simulink model "model_sysid_admittance"  (R2016b)
settings: Solver=FixedStepDiscrete  StartTime=0.0  StopTime=inf  FixedStep=sampleTime  RelTol=1e-3
PostLoadFcn:
  | % load model parameters
  | % pname = fileparts(get_param('model_base_bros','filename'));
  | % run([pname  '\parameters_base_model_bros.m']);
  | parameters_sysid_admittance;
  | 
  | % set requested state
  | set_param('model_sysid_admittance/Requested state','Value',num2str(0));
InitFcn:
  | % load model parameters
  | % pname = fileparts(get_param('model_base_bros','filename'));
  | % run([pname  '\parameters_base_model_bros.m']);
  | parameters_sysid_admittance;
  | 
  | % set requested state
  | set_param('model_sysid_admittance/Requested state','Value',num2str(0));
StartFcn:
  | parameters_sysid_admittance;
  | 
  | % set requested state
  | set_param('model_sysid_admittance/Requested state','Value',num2str(0));
values from neighbouring files (symbols this model uses):
  Ax = [0.00153392997769 0.00153392997769 0.00153392997769 0.00153392997769 0.00153392997769 0.00153392997769 0.00153392997769 0.00153392997769 0.00153392997769 0.00153392997769 0.00153392997769 0.00153392997769 ... (25 elements, 25x1)]    [data_inputsignal_admittance_100Hz.mat]
  Ay = [0.00153392997769 0.00153392997769 0.00153392997769 0.00153392997769 0.00153392997769 0.00153392997769 0.00153392997769 0.00153392997769 0.00153392997769 0.00153392997769 0.00153392997769 0.00153392997769 ... (25 elements, 25x1)]    [data_inputsignal_admittance_100Hz.mat]
  Lb = 0.07    [model_affc_parameters.m]    (also in parameters_sysid.m; parameters_sysid_admittance.m)
  Lf = 0.238    [model_affc_parameters.m]    (also in parameters_sysid.m; parameters_sysid_admittance.m)
  Lu = 0.153    [model_affc_parameters.m]    (also in parameters_sysid.m; parameters_sysid_admittance.m)
  nx = [5 7 11 13 17 23 29 37 47 61 79 103 ... (25 elements, 25x1)]    [data_inputsignal_admittance_100Hz.mat]
  ny = [3 8 10 14 19 24 31 41 53 67 83 107 ... (25 elements, 25x1)]    [data_inputsignal_admittance_100Hz.mat]
  phx = [1.20009664335 1.06282811403 1.3892882876 -0.190948998613 4.36135308948 3.55125265665 -1.29943418487 -0.0100316069113 1.01892216761 0.472716168264 1.16765179672 3.48382334533 ... (25 elements, 25x1)]    [data_inputsignal_admittance_100Hz.mat]
  phy = [4.61290873425 3.09865303555 -1.33576318949 -0.454866147562 0.315570179572 -1.54269258334 1.9231806523 3.28701306913 -0.551495079422 2.37779557242 1.0737629469 -1.42157877686 ... (25 elements, 25x1)]    [data_inputsignal_admittance_100Hz.mat]
  sampleTime = 0.001    [model_affc_parameters.m]    (also in parameters_sysid.m; parameters_sysid_admittance.m)
  Tm = 12    [data_inputsignal.mat]    (also in data_inputsignal_100Hz.mat; data_inputsignal_100Hz_n40.mat; data_inputsignal_150Hz_n50.mat; data_inputsignal_50Hz.mat)
undefined symbols (not defined in the file or in its folder): BROS3
libraries: simulink x14, LibraryFM x7, VariousBlocksLibrary x6, simulink_extras x1
(part 2 of 2)

== system model_sysid_admittance/Robot1/DataFromEtherCAT/Calculate Arrange Joint and Op Space/forward kinematics1 ==
  JointPosition_rad : Inport  PortDimensions=[2 1]
  JointVelocity_rads : Inport  Port=2  PortDimensions=[2 1]
  JointAcceleration_rads2 : Inport  Port=3  PortDimensions=[2 1]
  Je : MATLAB Function  TreatAsAtomicUnit=on
  Jedot : MATLAB Function  TreatAsAtomicUnit=on
  Product : Product  Multiplication=Matrix(*)
  calculate xddot : MATLAB Function  TreatAsAtomicUnit=on
  forward kinematics : MATLAB Function  TreatAsAtomicUnit=on
  x : Outport
  xdot : Outport  Port=2
  xddot : Outport  Port=3
  J : Outport  Port=4
  Jdot : Outport  Port=5
  wires:
  JointPosition_rad/1 -> forward kinematics/1(q), Jedot/1(q), Je/1(q)
  Je/1(Je) -> calculate xddot/3(J), Product/1, J/1
  JointVelocity_rads/1 -> calculate xddot/2(qdot), Product/2, Jedot/2(qdot)
  Jedot/1(Jedot) -> calculate xddot/4(Jdot), Jdot/1
  Product/1 -> xdot/1
  forward kinematics/1(x) -> x/1
  calculate xddot/1(xddot) -> xddot/1
  JointAcceleration_rads2/1 -> calculate xddot/1(qddot)

== matlab function model_sysid_admittance/Experiment & Haptics1/Admittance3/MATLAB Function ==
  data: t input; p output; nx parameter; Ax parameter; phx parameter; v output; a output; Tm parameter; ny parameter; Ay parameter; phy parameter
function [p,v,a] = fcn(t, nx, Ax, phx, Tm, ny, Ay, phy)
%#codegen

dw = 2*pi/Tm;
wx = nx*dw;
wy = ny*dw;

x = sum(Ax.*sin(wx*t+phx));
y = sum(Ay.*sin(wy*t+phy));
xdot = sum(wx.*Ax.*cos(wx*t+phx));
ydot = sum(wy.*Ay.*cos(wy*t+phy));
xddot = sum(-wx.^2.*Ax.*sin(wx*t+phx));
yddot = sum(-wy.^2.*Ay.*sin(wy*t+phy));

p = [x;y];
v = [xdot;ydot];
a = [xddot;yddot];

== matlab function model_sysid_admittance/Robot1/DataFromEtherCAT/Calculate Arrange Joint and Op Space/Condition number ==
  data: J input; C output
function C = conditioning(J)
%#codegen

C = norm(J)*norm(pinv(J));

== matlab function model_sysid_admittance/Robot1/DataFromEtherCAT/Calculate Arrange Joint and Op Space/forward kinematics1/Je ==
  data: q input; Je output size=[2 2]; Lf parameter; Lu parameter; Lb parameter
function Je = Je( q, Lf, Lu, Lb)
%#codegen

% Calculate the Jacobian for this particular device configuration.
% Note that the function func_eq_Je needs to be in the libraries/kinematis_functions folder

% jacobians
Je = func_eq_Je(q(1),q(2),Lf,Lu,Lb);

== matlab function model_sysid_admittance/Robot1/DataFromEtherCAT/Calculate Arrange Joint and Op Space/forward kinematics1/Jedot ==
  data: q input; qdot input; Jedot output size=[2 2]; Lf parameter; Lu parameter; Lb parameter
function Jedot = Jedot( q, qdot, Lf, Lu, Lb)
%#codegen

% Calculate the time derivative of the Jacobian for this particular device configuration.
% Note that the function func_eq_Je needs to be in the libraries/kinematis_functions folder


% jacobians
Jedot = func_eq_Jedot(q(1),q(2),qdot(1),qdot(2),Lf,Lu,Lb);

== matlab function model_sysid_admittance/Robot1/DataFromEtherCAT/Calculate Arrange Joint and Op Space/forward kinematics1/calculate xddot ==
  data: qddot input; qdot input size=[2 1]; J input; xddot output size=[2 1]; Jdot input
function xddot = calc_xddot(qddot, qdot, J, Jdot)
%#codegen

xddot = J*qddot + Jdot*qdot;

== matlab function model_sysid_admittance/Robot1/DataFromEtherCAT/Calculate Arrange Joint and Op Space/forward kinematics/forward kinematics ==
  data: q input; x output size=[2 1]; Lf parameter; Lu parameter; Lb parameter
function x = FK(q, Lf, Lu, Lb)
%#codegen

% Calculate the endpoint position (forward kinematics)
% Note that the function func_eq_FK needs to be in the libraries/kinematis_functions folder


x = func_eq_FK(q(1),q(2),Lf,Lu,Lb);

== matlab function model_sysid_admittance/Robot1/DataFromEtherCAT/Calculate Arrange Joint and Op Space/forward kinematics1/forward kinematics ==
  data: q input; x output size=[2 1]; Lf parameter; Lu parameter; Lb parameter
function x = FK(q, Lf, Lu, Lb)
%#codegen

% Calculate the endpoint position (forward kinematics)
% Note that the function func_eq_FK needs to be in the libraries/kinematis_functions folder


x = func_eq_FK(q(1),q(2),Lf,Lu,Lb);

== matlab function model_sysid_admittance/Robot1/DataToEtherCAT/FTSensorError/MATLAB Function ==
  data: ForcesTorques input; e output; MaxForcesTorques input
function e = fcn(ForcesTorques, MaxForcesTorques)

% throw error when any of the forces/torques go over a max allowable value
if any(abs(ForcesTorques) > MaxForcesTorques) 
    e = 1;
else
    e = 0;
end

== matlab function model_sysid_admittance/Robot1/Controller_PD/PD + nonlin (op space)/invJ1 ==
  data: x input; J input; y output
function y = invJ(x,J)

y = J.'*x;

== matlab function model_sysid_admittance/Robot1/DataFromEtherCAT/Calculate Arrange Joint and Op Space/forward kinematics/Je ==
  data: q input; Je output size=[2 2]; Lf parameter; Lu parameter; Lb parameter
function Je = Je( q, Lf, Lu, Lb)
%#codegen

% Calculate the Jacobian for this particular device configuration.
% Note that the function func_eq_Je needs to be in the libraries/kinematis_functions folder

% jacobians
Je = func_eq_Je(q(1),q(2),Lf,Lu,Lb);

== matlab function model_sysid_admittance/Robot1/DataFromEtherCAT/Calculate Arrange Joint and Op Space/forward kinematics/Jedot ==
  data: q input; qdot input; Jedot output size=[2 2]; Lf parameter; Lu parameter; Lb parameter
function Jedot = Jedot( q, qdot, Lf, Lu, Lb)
%#codegen

% Calculate the time derivative of the Jacobian for this particular device configuration.
% Note that the function func_eq_Je needs to be in the libraries/kinematis_functions folder


% jacobians
Jedot = func_eq_Jedot(q(1),q(2),qdot(1),qdot(2),Lf,Lu,Lb);

== matlab function model_sysid_admittance/Robot1/DataFromEtherCAT/FTSensor_K6D27/CorrectOffset ==
  data: u_in input; u_out output; reset input; corrected output
function [u_out,corrected] = CorrectOffset(u_in,reset)
%#codegen

persistent data_ offset_ counter_ corrected_;
N = 1000;

% initialize
if isempty(data_)
    data_ = zeros(size(u_in,1), N);
    offset_ = zeros(size(u_in));
    counter_ = 1;
    corrected_ = 0;
end

if (counter_ <= N)
    data_(:,counter_) = u_in;
end

counter_ = counter_ + 1;
if reset
    counter_ = 1;
end

% calculate mean
if counter_ == N
    corrected_ = 1;
    offset_ = mean(data_,2);
end

corrected = corrected_;
u_out = u_in - offset_;

== matlab function model_sysid_admittance/Robot1/DataFromEtherCAT/Calculate Arrange Joint and Op Space/IK all joints ==
  data: x input; q_all output; Lf parameter; Lu parameter; Lb parameter
function q_all = IK_all(x,Lf,Lu,Lb)
%#codegen

q_all = func_eqs_IK_all(x(1),x(2),Lf,Lu,Lb);

if any(isnan(q_all)) || any(isinf(q_all))
    q_all = zeros(5,1);
end

== matlab function model_sysid_admittance/Robot1/DataFromEtherCAT/Calculate Arrange Joint and Op Space/forward kinematics/calculate xddot ==
  data: qddot input; qdot input size=[2 1]; J input; xddot output size=[2 1]; Jdot input
function xddot = calc_xddot(qddot, qdot, J, Jdot)
%#codegen

xddot = J*qddot + Jdot*qdot;

== matlab function model_sysid_admittance/Robot1/Controller_PD/PD + nonlin (op space)/nonlinear compensation ==
  data: J input; Jdot input; qdot input; tau output; RobotStruct parameter
function tau = n(J,Jdot,qdot,RobotStruct)
% mass matrix
phat = RobotStruct.DynModParams;

% select parameters
me = phat(3);
Fs1 = phat(4);
Fv1 = phat(5);
Fs2 = phat(6);
Fv2 = phat(7);

% % jacobians
% J = func_eq_Je(q(1),q(2),Lf,Lu,Lb);
% Jdot = func_eq_Jedot(q(1),q(2),qdot(1),qdot(2),Lf,Lu,Lb);

% calculate joint space mass matrix;
p = [me;Fs1;Fv1;Fs2;Fv2];

% psi 
Psi = [(J'*Jdot)*qdot [ssign(qdot(1)) qdot(1); 0 0] [0 0; ssign(qdot(2)) qdot(2)]];

% torque
tau = Psi*p;

function x = ssign(u,b)
%% x = ssign(u,b)
% soft sign
if nargin < 2
    b = 8;
end

x = 2./(1+exp(-b*u))-1;

== matlab function model_sysid_admittance/Robot1/DataToEtherCAT/CreateSingleErrorValue2/ErrorToPower2 ==
  data: u input; e output
function e = errorToPowerOf2(u)

e = (2.^(0:length(u)-1))*u;

== matlab function model_sysid_admittance/Robot1/DataToEtherCAT/CreateSingleErrorValue1/ErrorToPower2 ==
  data: u input; e output
function e = errorToPowerOf2(u)

e = (2.^(0:length(u)-1))*u;

== matlab function model_sysid_admittance/Robot1/DataFromEtherCAT/FTSensor_K6D27/SensorToOperationalSpace ==
  data: q_all input; Fs input; FTOpSpace output; transmatside input
function FTOpSpace = ForceSensorToOperationalSpace(q_all,Fs,transmatside)
%#codegen
q1 = q_all(1);
q2 = q_all(2);
q4 = q_all(4);
q5 = q_all(5);

% based on which arm the force sensor is connected
switch transmatside
    case 1
        alpha = pi-q2;   
        beta = q1+alpha-pi/2;
        R0 = rotmat(beta);
        R = blkdiag(R0,R0); % transform forces and moments
    case 2
        alpha = -(pi - q4);
        beta = q5+alpha-pi/2;
        R0 = rotmat(beta);
        R = blkdiag(R0,R0); % transform forces and moments
    otherwise
        R = eye(length(Fs));
end

% transform force
FTOpSpace = R*Fs;

function R = rotmat(q)

R = [cos(q) -sin(q) 0;...
      sin(q)  cos(q) 0;...
      0       0      1];

== matlab function model_sysid_admittance/Robot1/DataToEtherCAT/WorkspacePositionGuard/CheckInternalAngles ==
  data: theta input; angleError output
function angleError = checkInternalErrors(theta)
%#codegen


angleError = 0;
if any(theta([2 4]) >= 0.95*pi)
    angleError = 1;
end

== matlab function model_sysid_admittance/Robot1/DataToEtherCAT/WorkspacePositionGuard/EndpointPositionGuard ==
  data: correctState input; xe input; error output
function error = fcn(correctState, xe)
%#codegen


error = 0;

% only check workspace boundaries after homing state is done
if ~correctState 
    return; 
end

% x0 = 0;
% y0 = 0.2354;
% a = 0.11;
% b = 0.08;

% workspace (see design document)
x0 = 0;
y0 = 0.25024;
a = 0.1746;
b = 0.13;%0.1048;

% check if endpoint is outside a predefined ellipse
x = xe(1);
y = xe(2);

% workspace is defined as an ellipse
e = (x-x0)^2 / a^2 + (y-y0)^2 / b^2;

% if is larger than 1, the endpoint is outside the workspace
if e > 1
    error = 1;
end
